simulink model "dc_mli"  (R2023b)
settings: Solver=VariableStepAuto  StartTime=0.0  StopTime=0.1  MaxStep=1e-6  RelTol=1e-3
model workspace (MAT data in the model file):
  Cdc = 0.00047
  Rdc = 0.001
  carrier_freq = 450
libraries: spsSeriesRLCBranchLib x9, spsIGBTLib x8, spsDiodeLib x6, simulink x4, spsGroundLib x2, spsCurrentMeasurementLib x1, spsDCVoltageSourceLib x1, dspstat3 x1, spsTHDLib x1, spsVoltageMeasurementLib x1, sps_lib x1
settings Model: Creator=ixale  LastModifiedBy=ixale
settings DataIOCC: ReturnWorkspaceOutputs=off

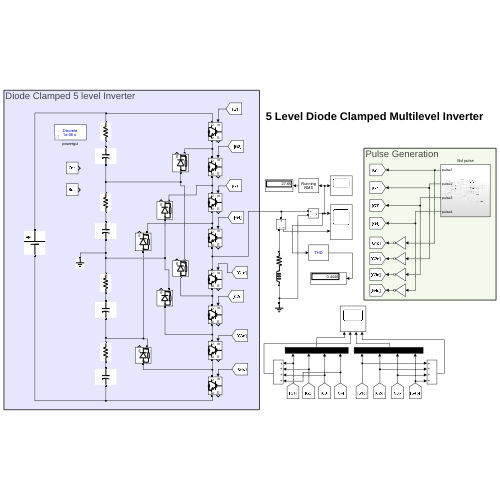
[thumbnail: Simulink's stored preview of the top-level diagram]
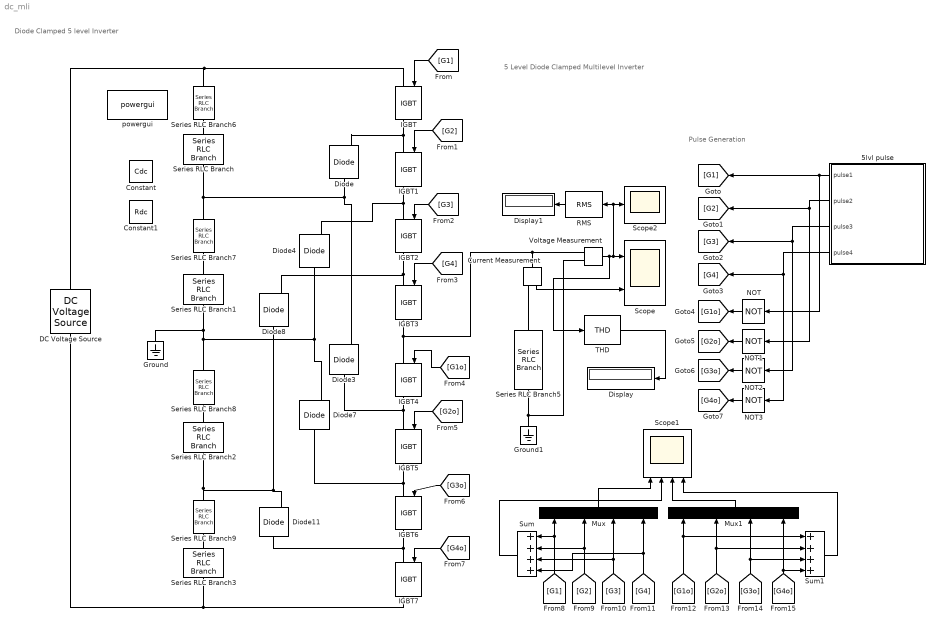
== system dc_mli ==
  note: Diode Clamped 5 level Inverter
  note: 5 Level Diode Clamped Multilevel Inverter
  note: Pulse Generation
  5lvl pulse : Subsystem
  Constant : Constant  Value=Cdc
  Constant1 : Constant  Value=Rdc
  Current Measurement : spsCurrentMeasurementLib/Current Measurement  PhasorSimulation=off  OutputType=Complex  PSBequivalent=0
  DC Voltage Source : spsDCVoltageSourceLib/DC Voltage Source  Amplitude=100  Measurements=None
  Diode{,3..4,7..8,11} (6 alike) : spsDiodeLib/Diode  Ron=0.001  Lon=0  Vf=0.8  IC=0  UseSnubber=0  Rs=500  Cs=250e-9  Measurements=on
  Display : Display
  Display1 : Display
  Ground : spsGroundLib/Ground  LConnTagsString=a
  Ground1 : spsGroundLib/Ground  LConnTagsString=a
  IGBT{,1..7} (8 alike) : spsIGBTLib/IGBT  Ron=0.001  Lon=0  Vf=1  Tf=1e-6  Tt=2e-6  IC=0  Rs=1e5  Cs=inf  Measurements=on
  Mux : Mux
  Mux1 : Mux
  NOT{,1..3} (4 alike) : Logic  Operator=NOT  IconShape=distinctive  AllPortsSameDT=off  OutDataTypeStr=boolean
  RMS : dspstat3/RMS  run=on  directionMode=Each column  dimension=1  InputProcessing=Columns as channels (frame based)  reset_popup=None
  Scope : Scope  NumInputPorts=2
  Scope1 : Scope  NumInputPorts=4
  Scope2 : Scope
  Series RLC Branch : spsSeriesRLCBranchLib/Series RLC Branch  LConnTagsString=__new0  RConnTagsString=__new0  BranchType=C  Resistance=1  Inductance=1e-3  SetiL0=off  InitialCurrent=0  Capacitance=Cdc  Setx0=off  InitialVoltage=0  Measurements=Branch voltage
  Series RLC Branch1 : spsSeriesRLCBranchLib/Series RLC Branch  LConnTagsString=__new0  RConnTagsString=__new0  BranchType=C  Resistance=1  Inductance=1e-3  SetiL0=off  InitialCurrent=0  Capacitance=Cdc  Setx0=off  InitialVoltage=0  Measurements=None
  Series RLC Branch2 : spsSeriesRLCBranchLib/Series RLC Branch  LConnTagsString=__new0  RConnTagsString=__new0  BranchType=C  Resistance=1  Inductance=1e-3  SetiL0=off  InitialCurrent=0  Capacitance=Cdc  Setx0=off  InitialVoltage=0  Measurements=Branch voltage
  Series RLC Branch3 : spsSeriesRLCBranchLib/Series RLC Branch  LConnTagsString=__new0  RConnTagsString=__new0  BranchType=C  Resistance=1  Inductance=1e-3  SetiL0=off  InitialCurrent=0  Capacitance=Cdc  Setx0=off  InitialVoltage=0  Measurements=Branch voltage
  Series RLC Branch5 : spsSeriesRLCBranchLib/Series RLC Branch  LConnTagsString=__new0  RConnTagsString=__new0  BranchType=RL  Resistance=100  Inductance=100e-3  SetiL0=off  InitialCurrent=0  Capacitance=10e-6  Setx0=off  InitialVoltage=0  Measurements=None
  Series RLC Branch{6..9} (4 alike) : spsSeriesRLCBranchLib/Series RLC Branch  LConnTagsString=__new0  RConnTagsString=__new0  BranchType=R  Resistance=Rdc  Inductance=1e-3  SetiL0=off  InitialCurrent=0  Capacitance=1e-6  Setx0=off  InitialVoltage=0  Measurements=None
  Sum : Sum  Inputs=++++
  Sum1 : Sum  Inputs=++++
  THD : spsTHDLib/THD  Freq=50  Ts=1e-6
  Voltage Measurement : spsVoltageMeasurementLib/Voltage Measurement  PhasorSimulation=off  OutputType=Complex  PSBequivalent=0
  powergui : sps_lib/powergui  Priority=1  SimulationMode=Discrete  SampleTime=1e-6  frequency=60  Iterations=50  frequencyindice=0  Pbase=100e6  ErrMax=1e-4  UnitsV=kV  UnitsW=MW  buscounter=0  FunctionMessages=off  echomessages=off  EnableUseOfTLC=off  CurrentSourceSwitches=off  DisableSnubberDevices=off  DisableRonSwitches=off  DisableVfSwitches=off  DisplayEquations=off  AutomaticDiscreteSolvers=off  SolverType=Tustin/Backward Euler (TBE)  Interpol=off  ExternalGateDelay=off  methode=off  Ts=100  x0status=blocks  SPID=on  SwTol=0  HookPort=off  NonlinearTolerance=1e-4  nMaxIteration=100  ContinueOnMaxIteration=off  RestoreLinks=warning  ResistiveCurrentMeasurement=off  Frange=[0:2:500]  Ylog=off  Xlog=on  ShowGrid=off  save=off  variable=ZData  structure=0  ZoomFFT=off  StartTime=0.0  cycles=1  DisplayStyle=1  fundamental=60  FreqAxis=off  MaxFrequency=1000  frequencyindicesteady=1  RmsSteady=1  display=off
  wires:
  5lvl pulse/1(pulse1) -> NOT/1, [G1]
  5lvl pulse/2(pulse2) -> NOT1/1, [G2]
  5lvl pulse/3(pulse3) -> NOT2/1, [G3]
  5lvl pulse/4(pulse4) -> NOT3/1, [G4]
  NOT/1 -> [G1o]
  NOT3/1 -> [G4o]
  NOT1/1 -> [G2o]
  [G1] -> IGBT/1
  [G2] -> IGBT1/1
  [G3] -> IGBT2/1
  [G4] -> IGBT3/1
  [G1o] -> IGBT4/1
  [G2o] -> IGBT5/1
  [G3o] -> IGBT6/1
  [G4o] -> IGBT7/1
  [G2] -> Mux/2, Sum/2
  [G1] -> Mux/1, Sum/1
  [G3] -> Sum/3, Mux/3
  [G4] -> Mux/4, Sum/4
  [G1o] -> Mux1/1, Sum1/1
  [G2o] -> Mux1/2, Sum1/2
  [G3o] -> Sum1/3, Mux1/3
  [G4o] -> Sum1/4, Mux1/4
  Sum/1 -> Scope1/2
  Sum1/1 -> Scope1/4
  NOT2/1 -> [G3o]
  Voltage Measurement/1 -> THD/1, RMS/1, Scope2/1, Scope/1
  Current Measurement/1 -> Scope/2
  THD/1 -> Display/1
  RMS/1 -> Display1/1
  Mux/1 -> Scope1/1
  Mux1/1 -> Scope1/3
  connections:
  Series RLC Branch6/RConn1 -- Series RLC Branch/LConn1
  IGBT/RConn1 -- Diode/RConn1 -- IGBT1/LConn1
  IGBT1/RConn1 -- Diode4/RConn1 -- IGBT2/LConn1
  IGBT2/RConn1 -- Diode8/RConn1 -- IGBT3/LConn1
  IGBT4/RConn1 -- Diode3/LConn1 -- IGBT5/LConn1
  IGBT5/RConn1 -- Diode7/LConn1 -- IGBT6/LConn1
  IGBT6/RConn1 -- Diode11/LConn1 -- IGBT7/LConn1
  IGBT3/RConn1 -- Current Measurement/LConn1 -- Voltage Measurement/LConn1 -- IGBT4/LConn1
  Series RLC Branch/RConn1 -- Series RLC Branch7/LConn1 -- Diode3/RConn1 -- Diode/LConn1
  Series RLC Branch2/RConn1 -- Series RLC Branch9/LConn1 -- Diode8/LConn1 -- Diode11/RConn1
  IGBT/LConn1 -- Series RLC Branch6/LConn1 -- DC Voltage Source/RConn1
  Ground/LConn1 -- Diode7/RConn1 -- Diode4/LConn1 -- Series RLC Branch8/LConn1 -- Series RLC Branch1/RConn1
  Series RLC Branch7/RConn1 -- Series RLC Branch1/LConn1
  Series RLC Branch8/RConn1 -- Series RLC Branch2/LConn1
  Series RLC Branch3/LConn1 -- Series RLC Branch9/RConn1
  IGBT7/RConn1 -- DC Voltage Source/LConn1 -- Series RLC Branch3/RConn1
  Ground1/LConn1 -- Voltage Measurement/LConn2 -- Series RLC Branch5/RConn1
  Current Measurement/RConn1 -- Series RLC Branch5/LConn1

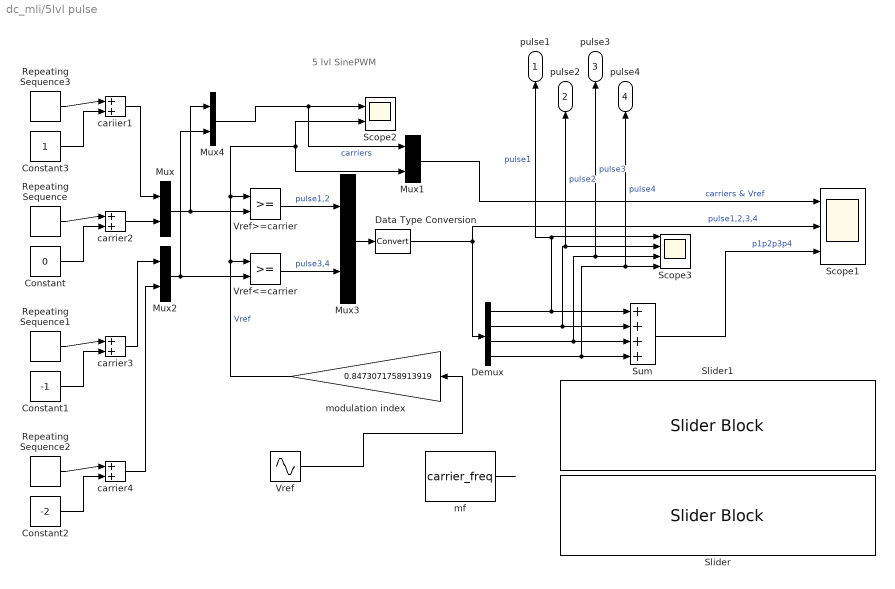
== system dc_mli/5lvl pulse ==
  note: 5 lvl SinePWM
  Constant : Constant  Value=0
  Constant1 : Constant  Value=-1
  Constant2 : Constant  Value=-2
  Constant3 : Constant
  Data Type Conversion : DataTypeConversion  SaturateOnIntegerOverflow=off  RndMeth=Floor
  Demux : Demux
  Mux{,1..4} (5 alike) : Mux  Inputs=2
  Repeating Sequence{,1..3} (4 alike) : simulink/Sources/Repeating Sequence  rep_seq_t=[0 0.5 1] / (50 * carrier_freq)  rep_seq_y=[0 1 0]
  Scope1 : Scope  NumInputPorts=3
  Scope2 : Scope  NumInputPorts=2
  Scope3 : Scope  NumInputPorts=4
  Slider : SliderBlock  ScaleMax=500
  Slider1 : SliderBlock  ScaleMax=1  TickInterval=0.1
  Sum : Sum  Inputs=++++
  Vref : Sin  Amplitude=2  Frequency=2*pi*50  SampleTime=0
  Vref<=carrier : RelationalOperator  OutDataTypeStr=boolean  RndMeth=Simplest  InputSameDT=off
  Vref>=carrier : RelationalOperator  OutDataTypeStr=boolean  RndMeth=Simplest  InputSameDT=off
  cariier1 : Sum  Inputs=|++
  carrier2 : Sum  Inputs=|++
  carrier3 : Sum  Inputs=|++
  carrier4 : Sum  Inputs=|++
  mf : Constant  Value=carrier_freq
  modulation index : Gain  Gain=0.8473071758913919
  pulse1 : Outport
  pulse2 : Outport  Port=2
  pulse3 : Outport  Port=3
  pulse4 : Outport  Port=4
  wires:
  Constant1/1 -> carrier3/2
  carrier2/1 -> Mux/2
  Constant3/1 -> cariier1/2
  Constant2/1 -> carrier4/2
  carrier4/1 -> Mux2/2
  Demux/1 -> pulse1/1, Scope3/1, Sum/1  "pulse1"
  Repeating Sequence3/1 -> cariier1/1
  Demux/4 -> Sum/4, pulse4/1, Scope3/4  "pulse4"
  Demux/3 -> pulse3/1, Scope3/3, Sum/3  "pulse3"
  modulation index/1 -> Scope2/2, Mux1/2, Vref>=carrier/1, Vref<=carrier/1  "Vref"
  Sum/1 -> Scope1/3  "p1p2p3p4"
  Repeating Sequence/1 -> carrier2/1
  Demux/2 -> Sum/2, pulse2/1, Scope3/2  "pulse2"
  cariier1/1 -> Mux/1
  Repeating Sequence2/1 -> carrier4/1
  Repeating Sequence1/1 -> carrier3/1
  mf/1 -> ?
  Mux1/1 -> Scope1/1  "carriers & Vref"
  carrier3/1 -> Mux2/1
  Vref/1 -> modulation index/1
  Constant/1 -> carrier2/2
  Mux3/1 -> Data Type Conversion/1
  Mux2/1 -> Vref<=carrier/2, Mux4/2
  Vref>=carrier/1 -> Mux3/1  "pulse1,2"
  Vref<=carrier/1 -> Mux3/2  "pulse3,4"
  Mux/1 -> Mux4/1, Vref>=carrier/2
  Data Type Conversion/1 -> Scope1/2, Demux/1  "pulse1,2,3,4"
  Mux4/1 -> Mux1/1, Scope2/1  "carriers"
